simulink library "outputCommands_ul"  (R2018b)
settings: Solver=VariableStepAuto  StartTime=0.0  StopTime=10.0  RelTol=1e-3
libraries: speedgoatlib_IO130 x2, simulink x1
settings Model: Creator=mcobb  LastModifiedBy=MAE-NCSUCORE
settings DebuggingCC: LibraryContextMissingDiagnostic=none
settings SFSimCC: SimUseLocalCustomCode=off
settings RTWCC: RTWUseLocalCustomCode=off

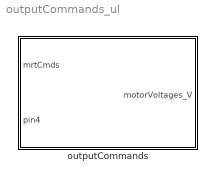
== system outputCommands_ul ==
  outputCommands : Subsystem  mask{maxVoltage=3.3}
      mask prompts: maxVoltage "Maximum Voltage [V]"
      mask help: Inputs are the commands from the 3 controllers. These are saturated to +/- 1 and then mapped to the entire voltage range specified by [0 MaxVoltage] where MaxVoltage is the user-specified quantity in the box below
      mask Display:
      | str_maxV = get_param(gcb,'maxVoltage');
      | 
      | if contains(str_maxV,'Value')
      |     dict = Simulink.data.dictionary.open('paramsDataDictionary.sldd');
      |     sect = getSection(dict,'Design Data');
      |     str = strsplit(str_maxV,'.');
      |     var = getEntry(sect,str{1});
      |     val = getValue(var);
      |     str = num2str(val.Value);
      | else
      |     str = str_maxV;
      | end
      | 
      | text(0.5, 0.8, [' \fontsize{12} \fontname{Cambria Math}Max Output \newline Voltage  ' str 'V'],...
      |     'horizontalAlignment', 'center','texmode','on')
      | 
      | port_label('input',1,'mtrCmds')
      | port_label('input',2,'pin4')
      | 
      | port_label('output',1,'motorVoltages_V')

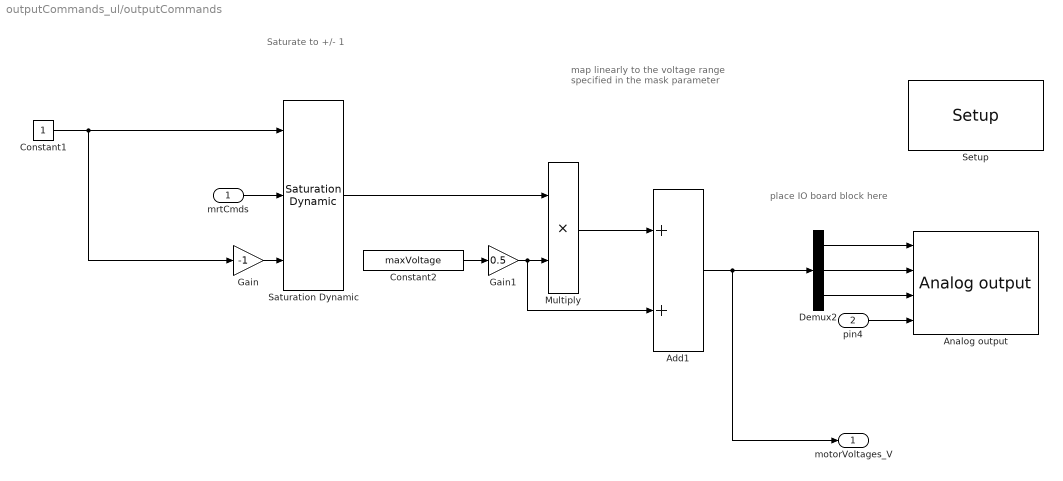
== system outputCommands_ul/outputCommands ==
  note: place IO board block here
  note: map linearly to the voltage range
      | specified in the mask parameter
  note: Saturate to +/- 1
  mrtCmds : Inport
  pin4 : Inport  Port=2
  Add1 : Sum
  "Analog output " : speedgoatlib_IO130/Analog output   parModuleId=1  parSampleTime=-1  parPciSlot=-1  parRange=+-5V  parChannels=[1 2 3 4]  parInitValues=[1.65 1.65 1.65 1.65]  parResetValues=[1 1 1 1]  parDmaChannels=All  parDmaEn=off  parDmaClkSrc=1  parDmaConversionTime=100  parDmaFrameSize=128  parBoardType=130  parDoInterrupt=on  parLatency=As small as possible  parIsInitialized=on
      settings: SourceProductName=Simulink Real-Time: Speedgoat I/O Driver Library
  Constant1 : Constant
  Constant2 : Constant  Value=maxVoltage
  Demux2 : Demux  Outputs=3
  Gain : Gain  Gain=-1
  Gain1 : Gain  Gain=0.5
  Multiply : Product
  Saturation Dynamic : simulink/Discontinuities/Saturation Dynamic  OutMin=[]  OutMax=[]  OutDataTypeStr=Inherit: Same as second input  OutDataType=fixdt(1, 16)  OutScaling=2^-10  DoSatur=off
  "Setup " : speedgoatlib_IO130/Setup   parPciSlot=-1  parModuleId=1  parTriggerInitiator=Independent  parAdChannels=1:8  parAdRange=+-5V  parAdOversampling=None  parAdContinuousSampling=off  parAdDmaEn=off  parAdDmaChannels=All  parAdSampleClock=100e3  parAdDmaFrameSize=128  parAdSampleTime=-1  parDaChannels=1:4  parDaRange=+-5V  parDaInitValues=[1.65]  parDaResetValues=[1]  parDaDmaEn=off  parDaDmaChannels=All  parLatency=As small as possible  parDaSampleClock=100000  parClockLocked=on  parDaDmaFrameSize=128  parDaSampleTime=-1  parBoardType=130  parForceRefresh=[]
      settings: SourceProductName=Simulink Real-Time: Speedgoat I/O Driver Library
  motorVoltages_V : Outport  LockScale=on
  wires:
  Constant1/1 -> Saturation Dynamic/1, Gain/1
  Gain/1 -> Saturation Dynamic/3
  Saturation Dynamic/1 -> Multiply/1
  Constant2/1 -> Gain1/1
  Multiply/1 -> Add1/1
  Gain1/1 -> Add1/2, Multiply/2
  Add1/1 -> motorVoltages_V/1, Demux2/1
  Demux2/3 -> "Analog output "/3
  Demux2/2 -> "Analog output "/2
  Demux2/1 -> "Analog output "/1
  pin4/1 -> "Analog output "/4
  mrtCmds/1 -> Saturation Dynamic/2
